simulink model "AudioEcho"  (R2015a)
settings: Solver=ode45  StartTime=0.0  StopTime=60  RelTol=1e-3
libraries: dsparch4 x2, simulink x1, dspvision x1, dspsnks4 x1
settings Model: Creator=ekulasek  LastModifiedBy=ekulasek

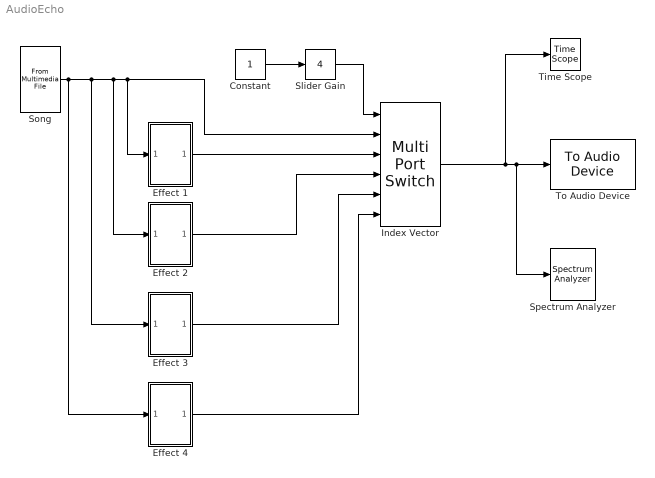
== system AudioEcho ==
  Constant : Constant
  Effect 1 : Subsystem
  Effect 2 : Subsystem
  Effect 3 : Subsystem
  Effect 4 : Subsystem
  Index Vector : MultiPortSwitch  DataPortOrder=Zero-based contiguous  Inputs=5  zeroidx=on
  Slider Gain : simulink/Math Operations/Slider Gain  low=0  gain=4  high=4
  Song : dspvision/From Multimedia File  inputFilename=/home/ekulasek/Malabe/classes/SignalsAndSystems/Programs/acappeller.wav  loop=on  numPlays=inf  outputStreams=Audio only  videoDataType=single  audioDataType=double  inheritSampleTime=on  userDefinedSampleTime=1/30  noAudioOutput=off  isIntensityVideo=off  fourcc=RGB  colorVideoFormat=Separate color signals  outputEOF=off  dataOrg=Column-major  audioFrameSize=1024  computeAudioFrameSize=off  outSamplingMode=Sample based
  Spectrum Analyzer : SpectrumAnalyzer
  Time Scope : TimeScope  DefaultConfigurationName=spbscopes.TimeScopeBlockCfg
  To Audio Device : dspsnks4/To Audio Device  deviceName=Default  inheritSampleRate=on  sampleRate=44100  deviceDatatype=Determine from input data type  autoBufferSize=on  bufferSize=4096  queueDuration=1.0  defaultOutputChannelMapping=on  outputChannelMapping=1:2  outputNumUnderrunSamples=off
  wires:
  Song/1 -> Effect 4/1(In1), Effect 3/1(In1), Effect 2/1(In1), Index Vector/2, Effect 1/1(In1)
  Effect 1/1(Out1) -> Index Vector/3
  Slider Gain/1 -> Index Vector/1
  Constant/1 -> Slider Gain/1
  Effect 2/1(Out1) -> Index Vector/4
  Index Vector/1 -> Time Scope/1, Spectrum Analyzer/1, To Audio Device/1
  Effect 3/1(Out1) -> Index Vector/5
  Effect 4/1(Out1) -> Index Vector/6

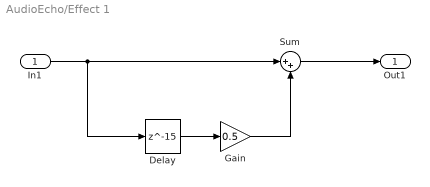
== system AudioEcho/Effect 1 ==
  In1 : Inport
  Delay : Delay  DelayLength=15  InitialCondition=0
  Gain : Gain  Gain=0.5
  Sum : Sum  Inputs=|++
  Out1 : Outport
  wires:
  Delay/1 -> Gain/1
  Sum/1 -> Out1/1
  Gain/1 -> Sum/2
  In1/1 -> Delay/1, Sum/1

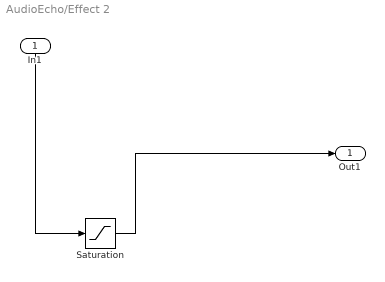
== system AudioEcho/Effect 2 ==
  In1 : Inport
  Saturation : Saturate  UpperLimit=0.15  LowerLimit=-0.15
  Out1 : Outport
  wires:
  Saturation/1 -> Out1/1
  In1/1 -> Saturation/1

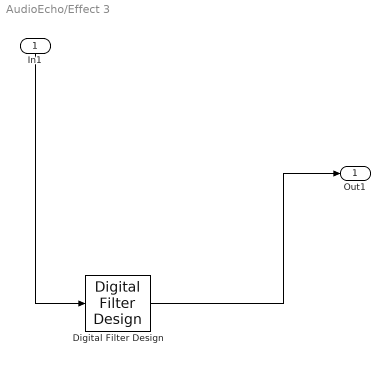
== system AudioEcho/Effect 3 ==
  In1 : Inport
  Digital Filter Design : dsparch4/Digital Filter Design  mwdsp_browser_bugfix_var=off
  Out1 : Outport
  wires:
  In1/1 -> Digital Filter Design/1
  Digital Filter Design/1 -> Out1/1

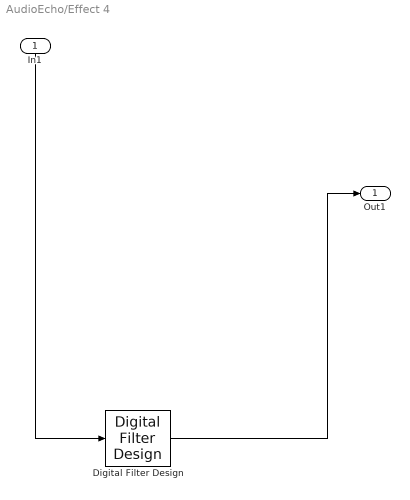
== system AudioEcho/Effect 4 ==
  In1 : Inport
  Digital Filter Design : dsparch4/Digital Filter Design  mwdsp_browser_bugfix_var=off
  Out1 : Outport
  wires:
  Digital Filter Design/1 -> Out1/1
  In1/1 -> Digital Filter Design/1
